simulink model "lab4"  (R2018a)
settings: Solver=VariableStepAuto  StartTime=0.0  StopTime=10.0  RelTol=1e-3
settings Model: Creator=Yan Tszyafen  LastModifiedBy=Yan Tszyafen

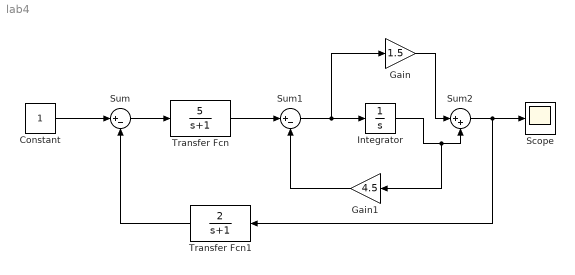
== system lab4 ==
  Constant : Constant
  Gain : Gain  Gain=1.5
  Gain1 : Gain  Gain=4.5
  Integrator : Integrator
  Scope : Scope
  Sum : Sum  Inputs=|+-
  Sum1 : Sum  Inputs=|+-
  Sum2 : Sum  Inputs=|++
  Transfer Fcn : TransferFcn  Numerator=[5]  Denominator=[1 1]
  Transfer Fcn1 : TransferFcn  Numerator=[2]  Denominator=[1 1]
  wires:
  Constant/1 -> Sum/1
  Transfer Fcn1/1 -> Sum/2
  Sum/1 -> Transfer Fcn/1
  Transfer Fcn/1 -> Sum1/1
  Gain1/1 -> Sum1/2
  Sum1/1 -> Gain/1, Integrator/1
  Integrator/1 -> Gain1/1, Sum2/2
  Gain/1 -> Sum2/1
  Sum2/1 -> Transfer Fcn1/1, Scope/1
